simulink model "FOC_Motor_Control"  (R2020b)
settings: Solver=FixedStepAuto  StartTime=0.0  StopTime=10.0  FixedStep=Fixed_Step_Size  RelTol=1e-3
undefined symbols (not defined in the file): Angle, Angle_offset, atan_table, Cosine_table, Dead_Com_Enable, Dead_Time, DiscIntNeverNeededParam, FF_Enable, Flux, FluxWeak_Enable, FluxWeak_Idref_max, FluxWeak_Idref_min, FluxWeak_Ki, FluxWeak_Kp, Harmonic_Com_Enable, Harmonic_Id5th_Ki, Harmonic_Id5th_Kp, Harmonic_Id5th_Max, Harmonic_Id5th_Min, Harmonic_Id7th_Ki, Harmonic_Id7th_Kp, Harmonic_Id7th_Max, Harmonic_Id7th_Min, Harmonic_Iq5th_Ki, Harmonic_Iq5th_Kp, Harmonic_Iq5th_Max, Harmonic_Iq5th_Min, Harmonic_Iq7th_Ki, Harmonic_Iq7th_Kp, Harmonic_Iq7th_Max, Harmonic_Iq7th_Min, ID_Ki, ID_Kp, inverter, IQ_Ki, IQ_Kp, LADRC_b0, LADRC_Omega_c, Ld, Lq, MTPA_id_table, MTPA_iq_table, MTPA_Te_Max, MTPA_Te_Min, Over_modulation, Pole_Pairs, PWM_Frequency, R, Sine_table, Speed_Ki, Speed_Kp, Speed_PI_OutputMax, Speed_PI_OutputMin, SpeedFilter_Fn, SVPWM, TorqueMode
libraries: simulink x6, powerlib_extras x4, pid_lib x1
(part 3 of 3)

== system FOC_Motor_Control/Motor_Control/Motor_Control_Function/FOC_Control_100us/FOC/Har_Compensation/Har_Compensation/idq57_Controller/I-park1 ==
  Ud7 : Inport
  Uq7 : Inport  Port=2
  Cos_theta : Inport  Port=3
  Sin_theta : Inport  Port=4
  Fcn : Fcn  Expr=u(1)*u(3)-u(2)*u(4)
  Fcn1 : Fcn  Expr=u(1)*u(4)+u(2)*u(3)
  Mux1 : Mux
  Ualfa7 : Outport  VectorParamsAs1DForOutWhenUnconnected=off
  Ubelt7 : Outport  Port=2  VectorParamsAs1DForOutWhenUnconnected=off
  wires:
  Ud7/1 -> Mux1/1
  Fcn/1 -> Ualfa7/1
  Mux1/1 -> Fcn1/1, Fcn/1
  Fcn1/1 -> Ubelt7/1
  Uq7/1 -> Mux1/2
  Cos_theta/1 -> Mux1/3
  Sin_theta/1 -> Mux1/4

== system FOC_Motor_Control/Motor_Control/Motor_Control_Function/FOC_Control_100us/FOC/Har_Compensation/Har_Compensation/idq57_Controller/ID_5 ==
  Err : Inport
  Add : Sum
  Discrete-Time Integrator : DiscreteIntegrator  SampleTime=-1  ICPrevOutput=DiscIntNeverNeededParam  ICPrevScaledInput=DiscIntNeverNeededParam
  Ki : Constant  Value=Harmonic_Id5th_Ki  OutDataTypeStr=single
  Kp : Constant  Value=Harmonic_Id5th_Kp  OutDataTypeStr=single
  Product : Product
  Product1 : Product
  Saturation : Saturate  UpperLimit=Harmonic_Id5th_Max  LowerLimit=Harmonic_Id5th_Min
  PI_Out : Outport
  wires:
  Kp/1 -> Product/1
  Err/1 -> Product1/2, Product/2
  Product1/1 -> Discrete-Time Integrator/1
  Product/1 -> Add/1
  Add/1 -> Saturation/1
  Saturation/1 -> PI_Out/1
  Discrete-Time Integrator/1 -> Add/2
  Ki/1 -> Product1/1

== system FOC_Motor_Control/Motor_Control/Motor_Control_Function/FOC_Control_100us/FOC/Har_Compensation/Har_Compensation/idq57_Controller/ID_7 ==
  Err : Inport
  Add : Sum
  Discrete-Time Integrator : DiscreteIntegrator  SampleTime=-1  ICPrevOutput=DiscIntNeverNeededParam  ICPrevScaledInput=DiscIntNeverNeededParam
  Ki : Constant  Value=Harmonic_Id7th_Ki  OutDataTypeStr=single
  Kp : Constant  Value=Harmonic_Id7th_Kp  OutDataTypeStr=single
  Product : Product
  Product1 : Product
  Saturation : Saturate  UpperLimit=Harmonic_Id7th_Max  LowerLimit=Harmonic_Id7th_Min
  PI_Out : Outport
  wires:
  Kp/1 -> Product/1
  Err/1 -> Product1/2, Product/2
  Product1/1 -> Discrete-Time Integrator/1
  Product/1 -> Add/1
  Add/1 -> Saturation/1
  Saturation/1 -> PI_Out/1
  Discrete-Time Integrator/1 -> Add/2
  Ki/1 -> Product1/1

== system FOC_Motor_Control/Motor_Control/Motor_Control_Function/FOC_Control_100us/FOC/Har_Compensation/Har_Compensation/idq57_Controller/IQ_5 ==
  Err : Inport
  Add : Sum
  Discrete-Time Integrator : DiscreteIntegrator  SampleTime=-1  ICPrevOutput=DiscIntNeverNeededParam  ICPrevScaledInput=DiscIntNeverNeededParam
  Ki : Constant  Value=Harmonic_Iq5th_Ki  OutDataTypeStr=single
  Kp : Constant  Value=Harmonic_Iq5th_Kp  OutDataTypeStr=single
  Product : Product
  Product1 : Product
  Saturation : Saturate  UpperLimit=Harmonic_Iq5th_Max  LowerLimit=Harmonic_Iq5th_Min
  PI_Out : Outport
  wires:
  Kp/1 -> Product/1
  Err/1 -> Product1/2, Product/2
  Product1/1 -> Discrete-Time Integrator/1
  Product/1 -> Add/1
  Add/1 -> Saturation/1
  Saturation/1 -> PI_Out/1
  Discrete-Time Integrator/1 -> Add/2
  Ki/1 -> Product1/1

== system FOC_Motor_Control/Motor_Control/Motor_Control_Function/FOC_Control_100us/FOC/Har_Compensation/Har_Compensation/idq57_Controller/IQ_7 ==
  Err : Inport
  Add : Sum
  Discrete-Time Integrator : DiscreteIntegrator  SampleTime=-1  ICPrevOutput=DiscIntNeverNeededParam  ICPrevScaledInput=DiscIntNeverNeededParam
  Ki : Constant  Value=Harmonic_Iq7th_Ki  OutDataTypeStr=single
  Kp : Constant  Value=Harmonic_Iq7th_Kp  OutDataTypeStr=single
  Product : Product
  Product1 : Product
  Saturation : Saturate  UpperLimit=Harmonic_Iq7th_Max  LowerLimit=Harmonic_Iq7th_Min
  PI_Out : Outport
  wires:
  Kp/1 -> Product/1
  Err/1 -> Product1/2, Product/2
  Product1/1 -> Discrete-Time Integrator/1
  Product/1 -> Add/1
  Add/1 -> Saturation/1
  Saturation/1 -> PI_Out/1
  Discrete-Time Integrator/1 -> Add/2
  Ki/1 -> Product1/1

== system FOC_Motor_Control/Motor_Control/Motor_Control_Function/FOC_Control_100us/FOC/Har_Compensation/Har_Compensation/idq57_Controller/Subsystem1 ==
  note: id
  note: we
  Id7 : Inport
  We : Inport  Port=2
  Iq7 : Inport  Port=3
  Fcn : Fcn  Expr=-u(2)*Lq*u(3)+R*u(1)
  Fcn1 : Fcn  Expr=u(2)*Ld*u(1)+R*u(3)
  Mux1 : Mux  Inputs=3
  Udc7 : Outport  VectorParamsAs1DForOutWhenUnconnected=off
  Uqc7 : Outport  Port=2  VectorParamsAs1DForOutWhenUnconnected=off
  wires:
  Iq7/1 -> Mux1/3
  Mux1/1 -> Fcn/1, Fcn1/1
  Fcn/1 -> Udc7/1
  We/1 -> Mux1/2
  Fcn1/1 -> Uqc7/1
  Id7/1 -> Mux1/1

== system FOC_Motor_Control/Motor_Control/Motor_Control_Function/FOC_Control_100us/FOC/Har_Compensation/Har_Compensation/idq57_Controller/Subsystem2 ==
  note: we
  note: id
  Id5 : Inport
  We : Inport  Port=2
  Iq5 : Inport  Port=3
  Fcn : Fcn  Expr=u(2)*Lq*u(3)+R*u(1)
  Fcn1 : Fcn  Expr=-u(2)*Ld*u(1)+R*u(3)
  Mux1 : Mux  Inputs=3
  Udc5 : Outport  VectorParamsAs1DForOutWhenUnconnected=off
  Uqc5 : Outport  Port=2  VectorParamsAs1DForOutWhenUnconnected=off
  wires:
  Id5/1 -> Mux1/1
  Fcn1/1 -> Uqc5/1
  We/1 -> Mux1/2
  Fcn/1 -> Udc5/1
  Mux1/1 -> Fcn/1, Fcn1/1
  Iq5/1 -> Mux1/3

== system FOC_Motor_Control/Motor_Control/Motor_Control_Function/FOC_Control_100us/FOC/DT_Compensation/DT_Compensation/IsTheta_Cal/Angle_calibration/If Action Subsystem1 ==
  Angle_input : Inport
  Action Port : ActionPort  ActionPortLabel=else
  Out1 : Outport
  wires:
  Angle_input/1 -> Out1/1

== system FOC_Motor_Control/Motor_Control/Motor_Control_Function/FOC_Control_100us/FOC/DT_Compensation/DT_Compensation/IsTheta_Cal/Angle_calibration/If Action Subsystem2 ==
  In1 : Inport
  Action Port : ActionPort  ActionPortLabel=if(u1 > 6.283185307)
  2pi : Constant  Value=2*pi  OutDataTypeStr=single
  Subtract1 : Sum  Inputs=+-
  Out1 : Outport
  wires:
  In1/1 -> Subtract1/1
  Subtract1/1 -> Out1/1
  2pi/1 -> Subtract1/2

== system FOC_Motor_Control/Motor_Control/Motor_Control_Function/FOC_Control_100us/FOC/DT_Compensation/DT_Compensation/IsTheta_Cal/atan/If Action Subsystem10 ==
  A_iq : Inport
  B_id : Inport  Port=2
  Action Port : ActionPort  ActionPortLabel=if((u1<0)&(u2<0))
  1-D Lookup Table4 : Lookup_n-D  NumberOfTableDimensions=1  LookupTableObject=''  BreakpointsForDimension1=single(linspace(-573,573,length(atan_table)));  BreakpointsForDimension1FirstPoint=10  BreakpointsForDimension2FirstPoint=10  BreakpointsForDimension1Spacing=12  BreakpointsForDimension2Spacing=12  IndexSearchMethod=Evenly spaced points  Table=atan_table  InterpMethod=Flat  DiagnosticForOutOfRangeInput=Error  InternalRulePriority=Speed  RndMeth=Simplest  InputSameDT=on
  Add : Sum  Inputs=+-
  Constant : Constant  Value=pi  OutDataTypeStr=single
  Divide : Product  Inputs=*/
  Saturation : Saturate  UpperLimit=572  LowerLimit=-572
  Scope : Scope
  IsTheta : Outport
  wires:
  Add/1 -> IsTheta/1
  Saturation/1 -> Scope/1, 1-D Lookup Table4/1
  A_iq/1 -> Divide/1
  Constant/1 -> Add/2
  Divide/1 -> Saturation/1
  B_id/1 -> Divide/2
  1-D Lookup Table4/1 -> Add/1

== system FOC_Motor_Control/Motor_Control/Motor_Control_Function/FOC_Control_100us/FOC/DT_Compensation/DT_Compensation/IsTheta_Cal/atan/If Action Subsystem11 ==
  Action Port : ActionPort  ActionPortLabel=if((u1>0)&(u2==0))
  Constant : Constant  Value=pi/2  OutDataTypeStr=single
  IsTheta : Outport
  wires:
  Constant/1 -> IsTheta/1

== system FOC_Motor_Control/Motor_Control/Motor_Control_Function/FOC_Control_100us/FOC/DT_Compensation/DT_Compensation/IsTheta_Cal/atan/If Action Subsystem12 ==
  Action Port : ActionPort  ActionPortLabel=if((u1<0)&(u2==0))
  Constant : Constant  Value=-pi/2  OutDataTypeStr=single
  IsTheta : Outport
  wires:
  Constant/1 -> IsTheta/1

== system FOC_Motor_Control/Motor_Control/Motor_Control_Function/FOC_Control_100us/FOC/DT_Compensation/DT_Compensation/IsTheta_Cal/atan/If Action Subsystem8 ==
  A_iq : Inport
  B_id : Inport  Port=2
  Action Port : ActionPort  ActionPortLabel=if((u1 >0))
  1-D Lookup Table4 : Lookup_n-D  NumberOfTableDimensions=1  LookupTableObject=''  BreakpointsForDimension1=single(linspace(-573,573,length(atan_table)));  BreakpointsForDimension1FirstPoint=10  BreakpointsForDimension2FirstPoint=10  BreakpointsForDimension1Spacing=12  BreakpointsForDimension2Spacing=12  IndexSearchMethod=Evenly spaced points  Table=atan_table  InterpMethod=Flat  DiagnosticForOutOfRangeInput=Error  InternalRulePriority=Speed  RndMeth=Simplest  InputSameDT=on
  Divide : Product  Inputs=*/
  Saturation : Saturate  UpperLimit=572  LowerLimit=-572
  Scope : Scope  NumInputPorts=2
  IsTheta : Outport
  wires:
  Divide/1 -> Saturation/1
  A_iq/1 -> Divide/1
  B_id/1 -> Divide/2
  Saturation/1 -> Scope/1, 1-D Lookup Table4/1
  1-D Lookup Table4/1 -> Scope/2, IsTheta/1

== system FOC_Motor_Control/Motor_Control/Motor_Control_Function/FOC_Control_100us/FOC/DT_Compensation/DT_Compensation/IsTheta_Cal/atan/If Action Subsystem9 ==
  A_iq : Inport
  B_id : Inport  Port=2
  Action Port : ActionPort  ActionPortLabel=if((u1>=0)&(u2<0))
  1-D Lookup Table4 : Lookup_n-D  NumberOfTableDimensions=1  LookupTableObject=''  BreakpointsForDimension1=single(linspace(-573,573,length(atan_table)));  BreakpointsForDimension1FirstPoint=10  BreakpointsForDimension2FirstPoint=10  BreakpointsForDimension1Spacing=12  BreakpointsForDimension2Spacing=12  IndexSearchMethod=Evenly spaced points  Table=atan_table  InterpMethod=Flat  DiagnosticForOutOfRangeInput=Error  InternalRulePriority=Speed  RndMeth=Simplest  InputSameDT=on
  Add : Sum
  Constant : Constant  Value=pi  OutDataTypeStr=single
  Divide : Product  Inputs=*/
  Saturation : Saturate  UpperLimit=572  LowerLimit=-572
  Scope : Scope  NumInputPorts=3
  IsTheta : Outport
  wires:
  B_id/1 -> Divide/2
  A_iq/1 -> Divide/1
  Add/1 -> Scope/3, IsTheta/1
  Constant/1 -> Add/2
  Saturation/1 -> Scope/1, 1-D Lookup Table4/1
  Divide/1 -> Saturation/1
  1-D Lookup Table4/1 -> Scope/2, Add/1
